simulink model "task9"  (R2019b)
settings: Solver=VariableStepAuto  StartTime=0.0  StopTime=20.0  MaxStep=1e-5  MinStep=1e-6  RelTol=1e-3
model workspace (MAT data in the model file):
  s = 0.6283185
undefined symbols (not defined in the file or in its folder): i
settings Model: Creator=misha  LastModifiedBy=misha
settings SolverCC: InitialStep=1e-6

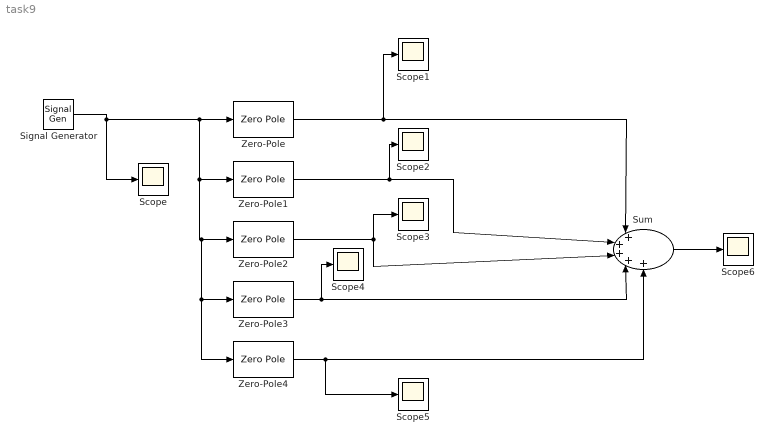
== system task9 ==
  Scope{,1..6} (7 alike) : Scope
  Signal Generator : SignalGenerator  WaveForm=square  Frequency=13
  Sum : Sum  Inputs=|+++++
  Zero-Pole : ZeroPole  Zeros=[0]  Poles=[-1 * 81.68 * 0.005 + i * 1 * 81.68 * 0.9999875, -1 * 81.68 * 0.005 - i * 1 * 81.68 * 0.9999875]  Gain=[1 * 81.68 * 0.01]
  Zero-Pole1 : ZeroPole  Zeros=[0]  Poles=[-2 * 81.68 * 0.005 + i * 2 * 81.68 * 0.9999875, -2 * 81.68 * 0.005 - i * 2 * 81.68 * 0.9999875]  Gain=[2 * 81.68 * 0.01]
  Zero-Pole2 : ZeroPole  Zeros=[0]  Poles=[-3 * 81.68 * 0.005 + i * 3 * 81.68 * 0.9999875, -3 * 81.68 * 0.005 - i * 3 * 81.68 * 0.9999875]  Gain=[3 * 81.68 * 0.01]
  Zero-Pole3 : ZeroPole  Zeros=[0]  Poles=[-4 * 81.68 * 0.005 + i * 4 * 81.68 * 0.9999875, -4 * 81.68 * 0.005 - i * 4 * 81.68 * 0.9999875]  Gain=[4 * 81.68 * 0.01]
  Zero-Pole4 : ZeroPole  Zeros=[0]  Poles=[-5 * 81.68 * 0.005 + i * 5 * 81.68 * 0.9999875, -5 * 81.68 * 0.005 - i * 5 * 81.68 * 0.9999875]  Gain=[5 * 81.68 * 0.01]
  wires:
  Signal Generator/1 -> Zero-Pole3/1, Zero-Pole4/1, Zero-Pole2/1, Zero-Pole1/1, Zero-Pole/1, Scope/1
  Zero-Pole/1 -> Scope1/1, Sum/1
  Zero-Pole1/1 -> Scope2/1, Sum/2
  Zero-Pole2/1 -> Scope3/1, Sum/3
  Zero-Pole3/1 -> Scope4/1, Sum/4
  Zero-Pole4/1 -> Scope5/1, Sum/5
  Sum/1 -> Scope6/1
